simulink model "threeDiskOscillatorRig_v4"  (R2024b)
settings: Solver=VariableStepAuto  StartTime=0.0  StopTime=simTime-6  RelTol=1e-3
values from neighbouring files (symbols this model uses):
  atan_scale = 100    [InputValues.m]    (also in threeDiskOscillator.m)
  b_1 = mean(ECP_values([6 7]))    [InputValues.m]    (also in threeDiskOscillator.m)
  b_2 = mean(ECP_values([8 9]))    [InputValues.m]    (also in threeDiskOscillator.m)
  b_3 = mean(ECP_values([10 11]))    [InputValues.m]    (also in threeDiskOscillator.m)
  C = [  1 0 0 0 0 0 ... (first row only)    [InputValues.m]    (also in threeDiskOscillator.m)
  C_aug = [C zeros(3,1)]    [threeDiskOscillator.m]
  F_aug = [F_d G_d(:,1);zeros(1,6) 1]    [threeDiskOscillator.m]
  f_m = [0;0;0]    [threeDiskOscillator.m]
  f_m_time = 8.5    [threeDiskOscillator.m]
  f_u = [0;-0.35]    [threeDiskOscillator.m]
  f_u_time = 25    [threeDiskOscillator.m]
  G_aug = [G_d;0 0]    [threeDiskOscillator.m]
  h = double(vpasolve(eq_1,gg))    [threeDiskOscillator.m]
  J_1 = ECP_values(1)    [InputValues.m]    (also in threeDiskOscillator.m)
  J_2 = ECP_values(2)    [InputValues.m]    (also in threeDiskOscillator.m)
  J_3 = ECP_values(3)    [InputValues.m]    (also in threeDiskOscillator.m)
  k_1 = ECP_values(4)    [InputValues.m]    (also in threeDiskOscillator.m)
  k_2 = ECP_values(5)    [InputValues.m]    (also in threeDiskOscillator.m)
  K_c = dlqr(F_d, G_d, Q_c, R_c)    [threeDiskOscillator.m]
  L_aug = dlqe(F_aug,eye(7),C_aug,1e-3*eye(7),sigma_meas(1,1).^2*eye(3))    [threeDiskOscillator.m]
  M_window = 20    [threeDiskOscillator.m]
  mu_0 = 0    [threeDiskOscillator.m]
  r1 = testout.r1.signals.values(:,1)    [threeDiskOscillator.m]
  r2 = testout.r1.signals.values(:,2)    [threeDiskOscillator.m]
  r3 = testout.r1.signals.values(:,3)    [threeDiskOscillator.m]
  sigma_meas = (0.0093^2)*eye(3)    [threeDiskOscillator.m]
  T_Cm = ECP_values(13)    [InputValues.m]    (also in threeDiskOscillator.m)
  T_Cp = ECP_values(12)    [InputValues.m]    (also in threeDiskOscillator.m)
  T_s = 4e-3    (= 0.004)    [threeDiskOscillator.m]
  w_th = 0.75    [InputValues.m]    (also in threeDiskOscillator.m)
  x_0 = [0;0;0;0;0;0]    [threeDiskOscillator.m]
undefined symbols (not defined in the file or in its folder): dspblkCoreblockFVToolHelper, gcbh, var
libraries: cstblocks x2, simulink x1
settings Model: Creator=nicol  LastModifiedBy=nicol

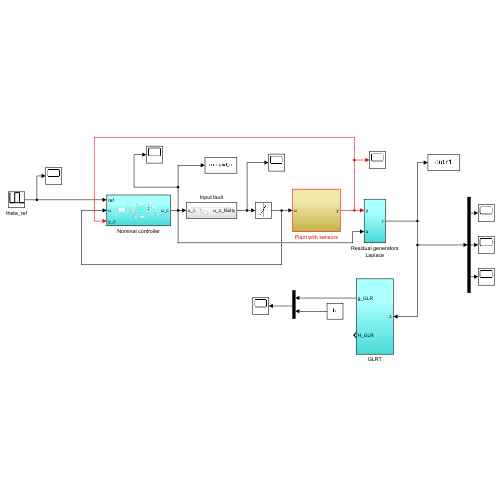
[thumbnail: Simulink's stored preview of the top-level diagram]
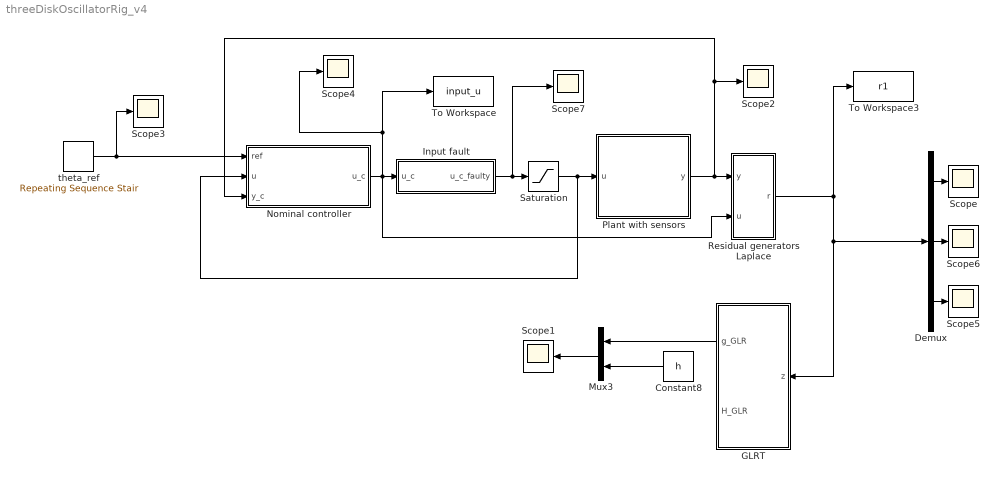
== system threeDiskOscillatorRig_v4 ==
  Constant8 : Constant  Value=h
  Demux : Demux  Outputs=3
  GLRT : Subsystem
  Input fault : Subsystem
  Mux3 : Mux  Inputs=2
  Nominal controller : Subsystem
  Plant with sensors : Subsystem
  Residual generators Laplace : Subsystem
  Saturation : Saturate  UpperLimit=2  LowerLimit=-2
  Scope{,1..7} (8 alike) : Scope
  To Workspace : ToWorkspace  VariableName=input_u  SaveFormat=Timeseries  SampleTime=T_s
  To Workspace3 : ToWorkspace  VariableName=r1  SaveFormat=Structure With Time  SampleTime=T_s
  theta_ref : simulink/Sources/Repeating Sequence Stair  OutValues=[0 1.57 0]  tsamp=5  OutMin=[]  OutMax=[]  OutDataTypeStr=double  OutputDataTypeScalingMode=double  OutDataType=fixdt(0,8)  ConRadixGroup=Best Precision: Vector-wise  OutScaling=2^-12
  wires:
  Constant8/1 -> Mux3/2
  Residual generators Laplace/1(r) -> Demux/1, GLRT/1(z), To Workspace3/1
  GLRT/1(g_GLR) -> Mux3/1
  Mux3/1 -> Scope1/1
  theta_ref/1 -> Scope3/1, Nominal controller/1(ref)
  Nominal controller/1(u_c) -> Residual generators Laplace/2(u), Scope4/1, To Workspace/1, Input fault/1(u_c)
  Input fault/1(u_c_faulty) -> Scope7/1, Saturation/1
  Plant with sensors/1(y) -> Scope2/1, Nominal controller/3(y_c), Residual generators Laplace/1(y)
  Saturation/1 -> Nominal controller/2(u), Plant with sensors/1(u)
  Demux/1 -> Scope/1
  Demux/3 -> Scope5/1
  Demux/2 -> Scope6/1

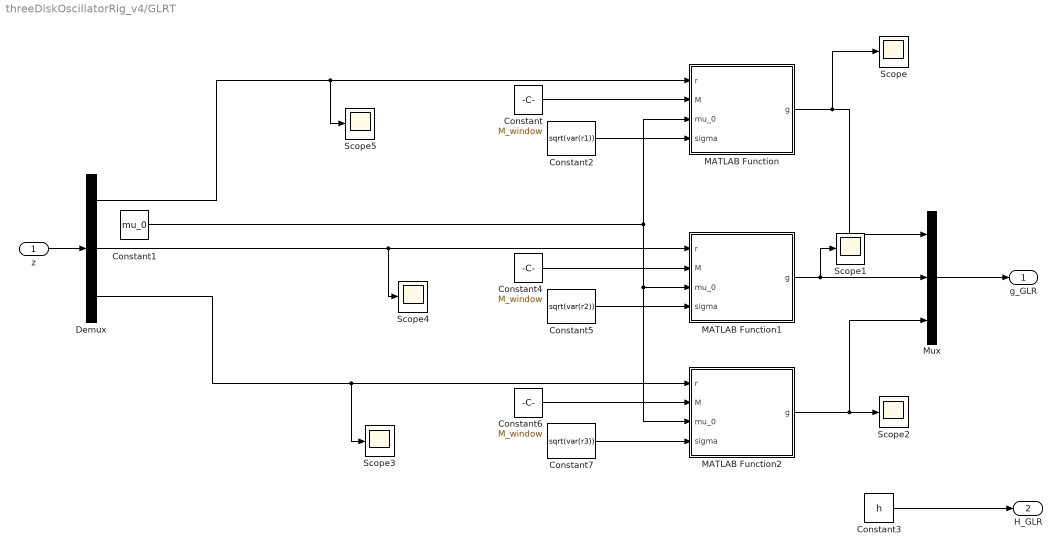
== system threeDiskOscillatorRig_v4/GLRT ==
  z : Inport
  Constant : Constant  Value=M_window
  Constant1 : Constant  Value=mu_0
  Constant2 : Constant  Value=sqrt(var(r1))
  Constant3 : Constant  Value=h
  Constant4 : Constant  Value=M_window
  Constant5 : Constant  Value=sqrt(var(r2))
  Constant6 : Constant  Value=M_window
  Constant7 : Constant  Value=sqrt(var(r3))
  Demux : Demux  Outputs=3
  MATLAB Function : MATLAB Function  TreatAsAtomicUnit=on
  MATLAB Function1 : MATLAB Function  TreatAsAtomicUnit=on
  MATLAB Function2 : MATLAB Function  TreatAsAtomicUnit=on
  Mux : Mux  Inputs=3
  Scope{,1..5} (6 alike) : Scope
  g_GLR : Outport  VectorParamsAs1DForOutWhenUnconnected=off
  H_GLR : Outport  Port=2  VectorParamsAs1DForOutWhenUnconnected=off
  wires:
  MATLAB Function/1(g) -> Scope/1, Mux/1
  Constant3/1 -> H_GLR/1
  z/1 -> Demux/1
  Demux/1 -> Scope5/1, MATLAB Function/1(r)
  Constant/1 -> MATLAB Function/2(M)
  Constant2/1 -> MATLAB Function/4(sigma)
  Constant4/1 -> MATLAB Function1/2(M)
  Constant5/1 -> MATLAB Function1/4(sigma)
  Demux/2 -> Scope4/1, MATLAB Function1/1(r)
  Demux/3 -> Scope3/1, MATLAB Function2/1(r)
  Constant7/1 -> MATLAB Function2/4(sigma)
  Constant6/1 -> MATLAB Function2/2(M)
  Constant1/1 -> MATLAB Function2/3(mu_0), MATLAB Function1/3(mu_0), MATLAB Function/3(mu_0)
  Mux/1 -> g_GLR/1
  MATLAB Function1/1(g) -> Scope1/1, Mux/2
  MATLAB Function2/1(g) -> Mux/3, Scope2/1

== system threeDiskOscillatorRig_v4/Input fault ==
  u_c : Inport
  Sum4 : Sum  Inputs=|++
  f_u : Step  Time=f_u_time  After=f_u  SampleTime=0
  u_c_faulty : Outport
  wires:
  f_u/1 -> Sum4/2
  u_c/1 -> Sum4/1
  Sum4/1 -> u_c_faulty/1

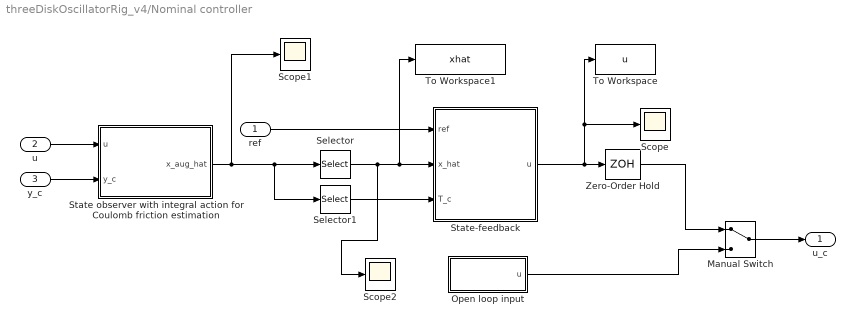
== system threeDiskOscillatorRig_v4/Nominal controller ==
  ref : Inport
  u : Inport  Port=2
  y_c : Inport  Port=3
  Manual Switch : ManualSwitch
  Open loop input : Subsystem
  Scope : Scope
  Scope1 : Scope
  Scope2 : Scope
  Selector : Selector  InputPortWidth=7  IndexOptions=Index vector (dialog)  Indices=[1:6]  OutputSizes=1
  Selector1 : Selector  InputPortWidth=7  IndexOptions=Index vector (dialog)  Indices=[7]  OutputSizes=1
  State observer with integral action for Coulomb friction estimation : Subsystem
  State-feedback : Subsystem
  To Workspace : ToWorkspace  VariableName=u  SaveFormat=Timeseries  SampleTime=T_s
  To Workspace1 : ToWorkspace  VariableName=xhat  SaveFormat=Structure  SampleTime=-1
  Zero-Order Hold : ZeroOrderHold  SampleTime=T_s
  u_c : Outport
  wires:
  Zero-Order Hold/1 -> Manual Switch/1
  y_c/1 -> State observer with integral action for Coulomb friction estimation/2(y_c)
  u/1 -> State observer with integral action for Coulomb friction estimation/1(u)
  Open loop input/1(u) -> Manual Switch/2
  Manual Switch/1 -> u_c/1
  Selector/1 -> Scope2/1, To Workspace1/1, State-feedback/2(x_hat)
  Selector1/1 -> State-feedback/3(T_c)
  State observer with integral action for Coulomb friction estimation/1(x_aug_hat) -> Scope1/1, Selector1/1, Selector/1
  ref/1 -> State-feedback/1(ref)
  State-feedback/1(u) -> To Workspace/1, Scope/1, Zero-Order Hold/1

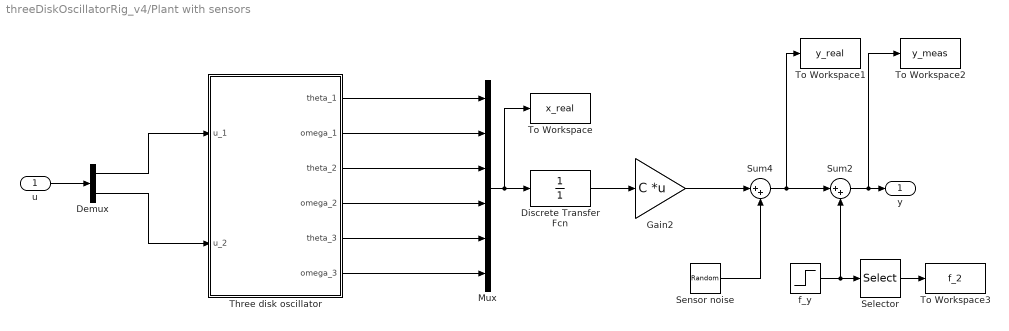
== system threeDiskOscillatorRig_v4/Plant with sensors ==
  u : Inport
  Demux : Demux  Outputs=2
  Discrete Transfer Fcn : DiscreteTransferFcn  LoadFcn=dspblkCoreblockFVToolHelper(gcbh,'load');  Denominator=[1]  SampleTime=T_s
      settings: CopyFcn=dspblkCoreblockFVToolHelper(gcbh,'copy');  DeleteFcn=dspblkCoreblockFVToolHelper(gcbh,'close');  ModelCloseFcn=dspblkCoreblockFVToolHelper(gcbh,'close');  PreSaveFcn=dspblkCoreblockFVToolHelper(gcbh,'presave');  PostSaveFcn=dspblkCoreblockFVToolHelper(gcbh,'postsave');  CloseFcn=dspblkCoreblockFVToolHelper(gcbh,'close');
  Gain2 : Gain  Gain=C  Multiplication=Matrix(K*u) (u vector)
  Mux : Mux  Inputs=6
  Selector : Selector  InputPortWidth=3  IndexOptions=Index vector (dialog)  Indices=[2]  OutputSizes=1
  Sensor noise : RandomNumber  Mean=zeros(3,1)  Variance=diag(sigma_meas^2)  SampleTime=T_s
  Sum2 : Sum  Inputs=|++
  Sum4 : Sum  Inputs=|++
  Three disk oscillator : Subsystem
  To Workspace : ToWorkspace  VariableName=x_real  SaveFormat=Timeseries  SampleTime=T_s
  To Workspace1 : ToWorkspace  VariableName=y_real  SaveFormat=Timeseries  SampleTime=T_s
  To Workspace2 : ToWorkspace  VariableName=y_meas  SaveFormat=Timeseries  SampleTime=T_s
  To Workspace3 : ToWorkspace  VariableName=f_2  SaveFormat=Timeseries  SampleTime=T_s
  f_y : Step  Time=f_m_time  Before=[0;0;0]  After=f_m  SampleTime=0
  y : Outport  VectorParamsAs1DForOutWhenUnconnected=off
  wires:
  u/1 -> Demux/1
  Three disk oscillator/2(omega_1) -> Mux/2
  Three disk oscillator/1(theta_1) -> Mux/1
  Mux/1 -> To Workspace/1, Discrete Transfer Fcn/1
  Three disk oscillator/4(omega_2) -> Mux/4
  Three disk oscillator/3(theta_2) -> Mux/3
  Discrete Transfer Fcn/1 -> Gain2/1
  Gain2/1 -> Sum4/1
  Sum4/1 -> To Workspace1/1, Sum2/1
  Sensor noise/1 -> Sum4/2
  Three disk oscillator/6(omega_3) -> Mux/6
  Three disk oscillator/5(theta_3) -> Mux/5
  f_y/1 -> Sum2/2, Selector/1
  Sum2/1 -> To Workspace2/1, y/1
  Selector/1 -> To Workspace3/1
  Demux/1 -> Three disk oscillator/1(u_1)
  Demux/2 -> Three disk oscillator/2(u_2)

== system threeDiskOscillatorRig_v4/Residual generators Laplace ==
  y : Inport
  u : Inport  Port=2
  LTI System : cstblocks/LTI System  sys=sys_y  IC=[]  PadeOrder=0
  LTI System1 : cstblocks/LTI System  sys=sys_u_normal  IC=[]  PadeOrder=0
  Sum : Sum  Inputs=|++
  r : Outport  VectorParamsAs1DForOutWhenUnconnected=off
  wires:
  Sum/1 -> r/1
  y/1 -> LTI System/1
  u/1 -> LTI System1/1
  LTI System/1 -> Sum/1
  LTI System1/1 -> Sum/2

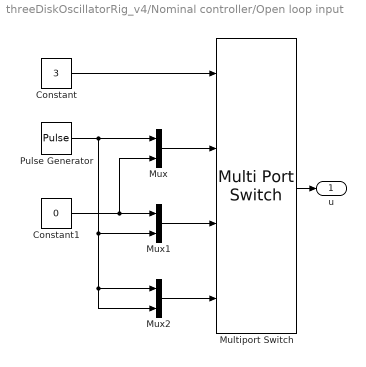
== system threeDiskOscillatorRig_v4/Nominal controller/Open loop input ==
  Constant : Constant  Value=3
  Constant1 : Constant  Value=0
  Multiport Switch : MultiPortSwitch  SaturateOnIntegerOverflow=off  InputSameDT=off
  Mux : Mux  Inputs=2
  Mux1 : Mux  Inputs=2
  Mux2 : Mux  Inputs=2
  Pulse Generator : DiscretePulseGenerator  PulseType=Time based  Period=10  PulseWidth=5
  u : Outport
  wires:
  Constant1/1 -> Mux1/1, Mux/2
  Pulse Generator/1 -> Mux2/2, Mux2/1, Mux1/2, Mux/1
  Constant/1 -> Multiport Switch/1
  Mux2/1 -> Multiport Switch/4
  Mux/1 -> Multiport Switch/2
  Multiport Switch/1 -> u/1
  Mux1/1 -> Multiport Switch/3

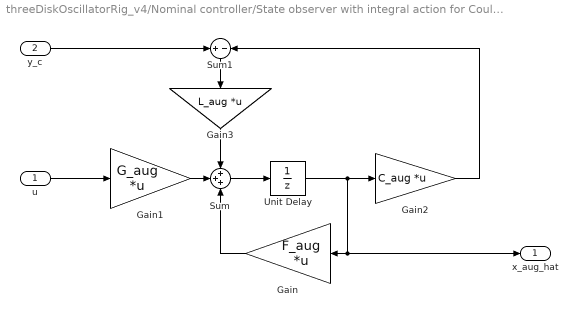
== system threeDiskOscillatorRig_v4/Nominal controller/State observer with integral action for Coulomb friction estimation ==
  u : Inport
  y_c : Inport  Port=2
  Gain : Gain  Gain=F_aug  Multiplication=Matrix(K*u) (u vector)
  Gain1 : Gain  Gain=G_aug  Multiplication=Matrix(K*u) (u vector)
  Gain2 : Gain  Gain=C_aug  Multiplication=Matrix(K*u) (u vector)
  Gain3 : Gain  Gain=L_aug  Multiplication=Matrix(K*u) (u vector)
  Sum : Sum  Inputs=+++
  Sum1 : Sum  Inputs=+-
  Unit Delay : UnitDelay  SampleTime=T_s  HasFrameUpgradeWarning=on
  x_aug_hat : Outport  VectorParamsAs1DForOutWhenUnconnected=off
  wires:
  Unit Delay/1 -> x_aug_hat/1, Gain/1, Gain2/1
  y_c/1 -> Sum1/1
  Sum1/1 -> Gain3/1
  Sum/1 -> Unit Delay/1
  Gain2/1 -> Sum1/2
  u/1 -> Gain1/1
  Gain1/1 -> Sum/2
  Gain/1 -> Sum/3
  Gain3/1 -> Sum/1

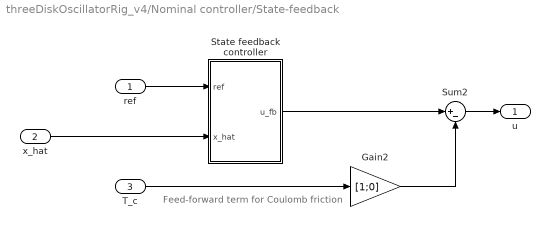
== system threeDiskOscillatorRig_v4/Nominal controller/State-feedback ==
  note: Feed-forward term for Coulomb friction
  ref : Inport
  x_hat : Inport  Port=2
  T_c : Inport  Port=3
  Gain2 : Gain  Gain=[1;0]
  State feedback controller : Subsystem
  Sum2 : Sum  Inputs=|+-
  u : Outport  VectorParamsAs1DForOutWhenUnconnected=off
  wires:
  T_c/1 -> Gain2/1
  Gain2/1 -> Sum2/2
  Sum2/1 -> u/1
  ref/1 -> State feedback controller/1(ref)
  x_hat/1 -> State feedback controller/2(x_hat)
  State feedback controller/1(u_fb) -> Sum2/1

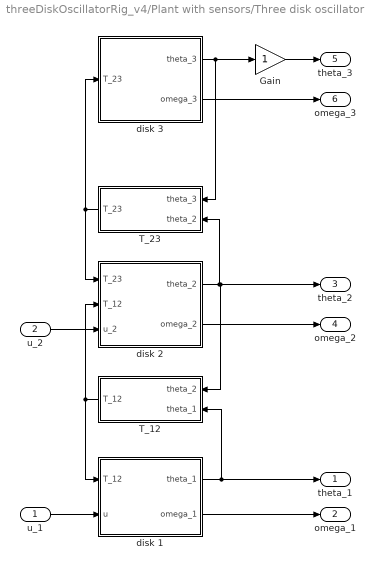
== system threeDiskOscillatorRig_v4/Plant with sensors/Three disk oscillator ==
  u_1 : Inport
  u_2 : Inport  Port=2
  Gain : Gain
  T_12 : Subsystem
  T_23 : Subsystem
  disk 1 : Subsystem
  disk 2 : Subsystem
  disk 3 : Subsystem
  theta_1 : Outport  VectorParamsAs1DForOutWhenUnconnected=off
  omega_1 : Outport  Port=2  VectorParamsAs1DForOutWhenUnconnected=off
  theta_2 : Outport  Port=3  VectorParamsAs1DForOutWhenUnconnected=off
  omega_2 : Outport  Port=4  VectorParamsAs1DForOutWhenUnconnected=off
  theta_3 : Outport  Port=5  VectorParamsAs1DForOutWhenUnconnected=off
  omega_3 : Outport  Port=6  VectorParamsAs1DForOutWhenUnconnected=off
  wires:
  T_23/1(T_23) -> disk 2/1(T_23), disk 3/1(T_23)
  disk 1/1(theta_1) -> T_12/2(theta_1), theta_1/1
  disk 2/1(theta_2) -> T_23/2(theta_2), theta_2/1, T_12/1(theta_2)
  T_12/1(T_12) -> disk 1/1(T_12), disk 2/2(T_12)
  disk 3/2(omega_3) -> omega_3/1
  disk 1/2(omega_1) -> omega_1/1
  disk 2/2(omega_2) -> omega_2/1
  u_1/1 -> disk 1/2(u)
  disk 3/1(theta_3) -> Gain/1, T_23/1(theta_3)
  Gain/1 -> theta_3/1
  u_2/1 -> disk 2/3(u_2)

== system threeDiskOscillatorRig_v4/Nominal controller/State-feedback/State feedback controller ==
  ref : Inport
  x_hat : Inport  Port=2
  Gain3 : Gain  Gain=K_c  Multiplication=Matrix(K*u) (u vector)
  Sum : Sum  Inputs=|+-
  u_fb : Outport
  wires:
  x_hat/1 -> Gain3/1
  ref/1 -> Sum/1
  Sum/1 -> u_fb/1
  Gain3/1 -> Sum/2

== system threeDiskOscillatorRig_v4/Plant with sensors/Three disk oscillator/T_12 ==
  theta_2 : Inport
  theta_1 : Inport  Port=2
  Gain : Gain  Gain=k_1
  Sum : Sum  Inputs=|+-
  T_12 : Outport  VectorParamsAs1DForOutWhenUnconnected=off
  wires:
  theta_2/1 -> Sum/2
  theta_1/1 -> Sum/1
  Sum/1 -> Gain/1
  Gain/1 -> T_12/1

== system threeDiskOscillatorRig_v4/Plant with sensors/Three disk oscillator/T_23 ==
  theta_3 : Inport
  theta_2 : Inport  Port=2
  Gain : Gain  Gain=k_2
  Sum : Sum  Inputs=-+|
  T_23 : Outport  VectorParamsAs1DForOutWhenUnconnected=off
  wires:
  Gain/1 -> T_23/1
  Sum/1 -> Gain/1
  theta_3/1 -> Sum/1
  theta_2/1 -> Sum/2

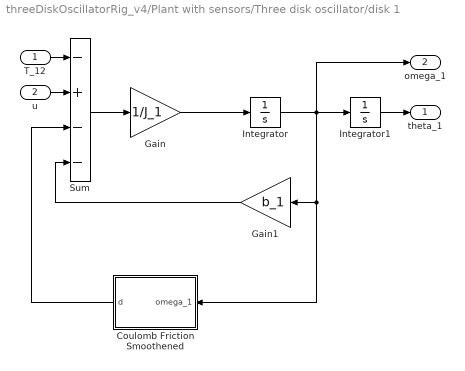
== system threeDiskOscillatorRig_v4/Plant with sensors/Three disk oscillator/disk 1 ==
  T_12 : Inport
  u : Inport  Port=2
  Coulomb Friction Smoothened : Subsystem
  Gain : Gain  Gain=1/J_1
  Gain1 : Gain  Gain=b_1
  Integrator : Integrator  InitialCondition=x_0(2)
  Integrator1 : Integrator  InitialCondition=x_0(1)
  Sum : Sum  Inputs=-+--
  theta_1 : Outport  VectorParamsAs1DForOutWhenUnconnected=off
  omega_1 : Outport  Port=2  VectorParamsAs1DForOutWhenUnconnected=off
  wires:
  Sum/1 -> Gain/1
  Integrator/1 -> Integrator1/1, omega_1/1, Coulomb Friction Smoothened/1(omega_1), Gain1/1
  Gain1/1 -> Sum/4
  Integrator1/1 -> theta_1/1
  T_12/1 -> Sum/1
  u/1 -> Sum/2
  Gain/1 -> Integrator/1
  Coulomb Friction Smoothened/1(d) -> Sum/3

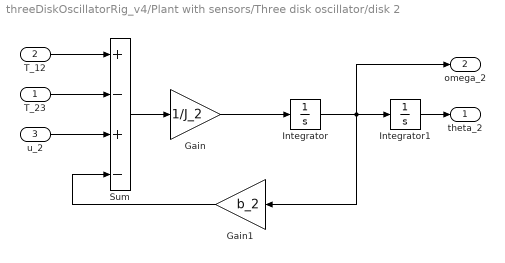
== system threeDiskOscillatorRig_v4/Plant with sensors/Three disk oscillator/disk 2 ==
  T_23 : Inport
  T_12 : Inport  Port=2
  u_2 : Inport  Port=3
  Gain : Gain  Gain=1/J_2
  Gain1 : Gain  Gain=b_2
  Integrator : Integrator  InitialCondition=x_0(4)
  Integrator1 : Integrator  InitialCondition=x_0(3)
  Sum : Sum  Inputs=+-+-
  theta_2 : Outport  VectorParamsAs1DForOutWhenUnconnected=off
  omega_2 : Outport  Port=2  VectorParamsAs1DForOutWhenUnconnected=off
  wires:
  T_23/1 -> Sum/2
  T_12/1 -> Sum/1
  Integrator1/1 -> theta_2/1
  Gain1/1 -> Sum/4
  Gain/1 -> Integrator/1
  Integrator/1 -> Integrator1/1, Gain1/1, omega_2/1
  Sum/1 -> Gain/1
  u_2/1 -> Sum/3

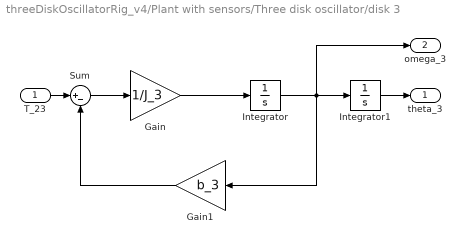
== system threeDiskOscillatorRig_v4/Plant with sensors/Three disk oscillator/disk 3 ==
  T_23 : Inport
  Gain : Gain  Gain=1/J_3
  Gain1 : Gain  Gain=b_3
  Integrator : Integrator  InitialCondition=x_0(6)
  Integrator1 : Integrator  InitialCondition=x_0(5)
  Sum : Sum  Inputs=|+-
  theta_3 : Outport  VectorParamsAs1DForOutWhenUnconnected=off
  omega_3 : Outport  Port=2  VectorParamsAs1DForOutWhenUnconnected=off
  wires:
  Sum/1 -> Gain/1
  Integrator/1 -> Integrator1/1, omega_3/1, Gain1/1
  Gain/1 -> Integrator/1
  Gain1/1 -> Sum/2
  Integrator1/1 -> theta_3/1
  T_23/1 -> Sum/1

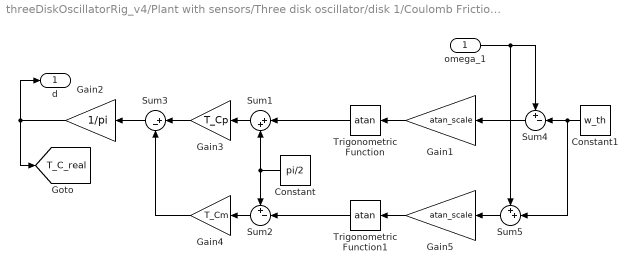
== system threeDiskOscillatorRig_v4/Plant with sensors/Three disk oscillator/disk 1/Coulomb Friction Smoothened ==
  omega_1 : Inport
  Constant : Constant  Value=pi/2
  Constant1 : Constant  Value=w_th
  Gain1 : Gain  Gain=atan_scale
  Gain2 : Gain  Gain=1/pi
  Gain3 : Gain  Gain=T_Cp
  Gain4 : Gain  Gain=T_Cm
  Gain5 : Gain  Gain=atan_scale
  Sum1 : Sum  Inputs=|++
  Sum2 : Sum  Inputs=+-|
  Sum3 : Sum  Inputs=|+-
  Sum4 : Sum  Inputs=+-|
  Sum5 : Sum  Inputs=++|
  Trigonometric Function : Trigonometry  Operator=atan
  Trigonometric Function1 : Trigonometry  Operator=atan
  d : Outport  VectorParamsAs1DForOutWhenUnconnected=off
  tag scope: T_C_real=global
  wires:
  Gain1/1 -> Trigonometric Function/1
  Sum1/1 -> Gain3/1
  Constant/1 -> Sum2/1, Sum1/2
  Sum2/1 -> Gain4/1
  Sum3/1 -> Gain2/1
  Trigonometric Function/1 -> Sum1/1
  Gain4/1 -> Sum3/2
  Gain2/1 -> [T_C_real], d/1
  omega_1/1 -> Sum5/1, Sum4/1
  Gain3/1 -> Sum3/1
  Sum4/1 -> Gain1/1
  Constant1/1 -> Sum5/2, Sum4/2
  Gain5/1 -> Trigonometric Function1/1
  Sum5/1 -> Gain5/1
  Trigonometric Function1/1 -> Sum2/2

== matlab function threeDiskOscillatorRig_v4/GLRT/MATLAB Function1 ==
  settings: updateMethod=DISCRETE
  data: r input; M input; mu_0 input; sigma input; g output
function g  = GLR(r,M,mu_0,sigma)
%GLR 
%M =initial guess of window size
%mu_0 = mean value when no fault occured 
%sigma = standard deviation of residual

  persistent buffer mu_1 idx
  g = 0;
 
 %initialization at start
 if (isempty(buffer))
    buffer = zeros(1, M);
    %g = 0;      
    mu_1 = 0;   
    idx = 0;    
 end

%right shift buffer which keeps the lates M samples: 
buffer = [r, buffer(1:end-1)];   
if length(buffer) > M
    buffer = buffer(1:M);
end

% Compute GLR When M samples are stores in the buffer
if (length(buffer) == M)
    S = zeros(M, 1);  % Define the log-likelihood ratio
    z = buffer;       % extract the residual samples inside the window 
    for j = 1:M       % Iterate for all the time instants of the window
        sum_sq = 0;
        for i = j:M
            sum_sq = sum_sq + (z(i) - mu_0);
        end
        S(j) = sum_sq^2 / ((M - j + 1) * 2 * sigma^2);
    end
    
    % Find maximum GLR statistic and corresponding index
    [g, idx] = max(S); 
    mu_1= sum(buffer(idx:end)) / (M - idx + 1);
else 
    j=0
    z=buffer;
    sum_sq=0;
    S = zeros(M, 1); 

end

end

== matlab function threeDiskOscillatorRig_v4/GLRT/MATLAB Function ==
  settings: updateMethod=DISCRETE
  data: r input; M input; mu_0 input; sigma input; g output
function g  = GLR(r,M,mu_0,sigma)
%GLR 
%M =initial guess of window size
%mu_0 = mean value when no fault occured 
%sigma = standard deviation of residual

  persistent buffer mu_1 idx
  g = 0;
 
 %initialization at start
 if (isempty(buffer))
    buffer = zeros(1, M);
    %g = 0;      
    mu_1 = 0;   
    idx = 0;    
 end

%right shift buffer which keeps the lates M samples: 
buffer = [r, buffer(1:end-1)];   
if length(buffer) > M
    buffer = buffer(1:M);
end

% Compute GLR When M samples are stores in the buffer
if (length(buffer) == M)
    S = zeros(M, 1);  % Define the log-likelihood ratio
    z = buffer;       % extract the residual samples inside the window 
    for j = 1:M       % Iterate for all the time instants of the window
        sum_sq = 0;
        for i = j:M
            sum_sq = sum_sq + (z(i) - mu_0);
        end
        S(j) = sum_sq^2 / ((M - j + 1) * 2 * sigma^2);
    end
    
    % Find maximum GLR statistic and corresponding index
    [g, idx] = max(S); 
    mu_1= sum(buffer(idx:end)) / (M - idx + 1);
else 
    j=0
    z=buffer;
    sum_sq=0;
    S = zeros(M, 1); 

end

end

== matlab function threeDiskOscillatorRig_v4/GLRT/MATLAB Function2 ==
  settings: updateMethod=DISCRETE
  data: r input; M input; mu_0 input; sigma input; g output
function g  = GLR(r,M,mu_0,sigma)
%GLR 
%M =initial guess of window size
%mu_0 = mean value when no fault occured 
%sigma = standard deviation of residual

  persistent buffer mu_1 idx
  g = 0;
 
 %initialization at start
 if (isempty(buffer))
    buffer = zeros(1, M);
    %g = 0;      
    mu_1 = 0;   
    idx = 0;    
 end

%right shift buffer which keeps the lates M samples: 
buffer = [r, buffer(1:end-1)];   
if length(buffer) > M
    buffer = buffer(1:M);
end

% Compute GLR When M samples are stores in the buffer
if (length(buffer) == M)
    S = zeros(M, 1);  % Define the log-likelihood ratio
    z = buffer;       % extract the residual samples inside the window 
    for j = 1:M       % Iterate for all the time instants of the window
        sum_sq = 0;
        for i = j:M
            sum_sq = sum_sq + (z(i) - mu_0);
        end
        S(j) = sum_sq^2 / ((M - j + 1) * 2 * sigma^2);
    end
    
    % Find maximum GLR statistic and corresponding index
    [g, idx] = max(S); 
    mu_1= sum(buffer(idx:end)) / (M - idx + 1);
else 
    j=0
    z=buffer;
    sum_sq=0;
    S = zeros(M, 1); 

end

end
